simulink model "transmitter"  (R2020b)
settings: Solver=FixedStepDiscrete  StartTime=0.0  StopTime=100000  RelTol=1e-3
undefined symbols (not defined in the file): message
libraries: hdlsllib x24, simulink x11, dspmlti4 x2, whdlio x1
(part 2 of 2)

== matlab function transmitter/tran_dut/ldpc_encoder/address_calculator/addresses ==
  settings: fimath=fimath('RoundingMethod', 'Floor','OverflowAction', 'Wrap','ProductMode', 'FullPrecision', 'SumMode', 'FullPrecision')
  data: slot input; counter input; q_factor input; addresses output; bit_addresses parameter uint16; num_parity_bits parameter
function addresses = address_generator(slot, counter, q_factor, bit_addresses, num_parity_bits)
%#codegen 

addresses = fi(zeros(12, 1), 0, 14, 0);

coder.hdl.loopspec('unroll');
% Get the new parity address
for i = 1:12
    tmp = fi(16200, 0, 15, 0);
    if bit_addresses(slot, i) < 16200
        % Compute the new address
        tmp = fi(bit_addresses(slot, i) + counter*q_factor, 0, 15, 0);
        % Get the modulo 16200 if necessary.
        if tmp >= num_parity_bits
            tmp = fi(tmp - num_parity_bits, 0, 15, 0);
        end
    end
    addresses(i) = fi(tmp, 0, 14, 0);
end

== matlab function transmitter/tran_dut/ldpc_encoder/select_address ==
  settings: fimath=fimath('RoundingMethod', 'Floor','OverflowAction', 'Wrap','ProductMode', 'FullPrecision', 'SumMode', 'FullPrecision')
  data: addresses input; a1 output; a2 output; a3 output; a4 output; a5 output; a6 output; a7 output; a8 output; a9 output; a10 output; a11 output; a12 output
function [a1,a2,a3,a4,a5,a6,...
          a7,a8,a9,a10,a11,a12] = select(addresses)
%#codegen

a1 = addresses(1);
a2 = addresses(2);
a3 = addresses(3);
a4 = addresses(4);
a5 = addresses(5);
a6 = addresses(6);
a7 = addresses(7);
a8 = addresses(8);
a9 = addresses(9);
a10 = addresses(10);
a11 = addresses(11);
a12 = addresses(12);

== matlab function transmitter/tran_dut/bch_encoder/output_mask ==
  settings: fimath=fimath('RoundingMethod', 'Floor','OverflowAction', 'Wrap','ProductMode', 'FullPrecision', 'SumMode', 'FullPrecision')
  data: bit_in input; mask output
function mask = bitmask(bit_in)
%#codegen

if bit_in
    mask = fi(ones(192, 1), 0, 1, 0);
else
    mask = fi(zeros(192, 1), 0, 1, 0);
end

== matlab function transmitter/tran_dut/bch_encoder/p2s ==
  settings: fimath=fimath('RoundingMethod', 'Floor','OverflowAction', 'Wrap','ProductMode', 'FullPrecision', 'SumMode', 'FullPrecision')
  data: parallel_in input; serial_out output fixdt(0,1,0); enable input; input_length parameter uint16; valid output
function [serial_out, valid] = p2s_buffer(parallel_in, enable, input_length)
%#codegen

state_iddle    = 0;
state_reading  = 1;

persistent moore_state_machine;
if isempty(moore_state_machine)
    moore_state_machine = fi(0, 0, 1, 0);
end

persistent counter;
if isempty(counter)
    counter = fi(1, 0, 16, 0);
end

persistent buffer;
if isempty(buffer)
    buffer = parallel_in;
end

switch moore_state_machine
    case state_iddle
        serial_out = fi(0, 0, 1, 0);
        valid      = fi(0, 0, 1, 0);
        if enable
            moore_state_machine(1) = state_reading;
            buffer = parallel_in;
            serial_out          = buffer(input_length+1-counter);
            valid      = fi(1, 0, 1, 0);
            counter             = fi(counter + 1, 0, 16, 0);
        end
    case state_reading
        serial_out = buffer(input_length+1-counter);
        counter    = fi(counter + 1, 0, 16, 0);
        valid      = fi(1, 0, 1, 0);
        if(counter > input_length)
            counter = fi(1, 0, 16, 0);
            moore_state_machine(1) = state_iddle;
        end
    otherwise
        serial_out = fi(0, 0, 1, 0);
        valid      = fi(0, 0, 1, 0);
end

== matlab function transmitter/tran_dut/bch_encoder/registers ==
  settings: fimath=fimath('RoundingMethod', 'Floor','OverflowAction', 'Wrap','ProductMode', 'FullPrecision', 'SumMode', 'FullPrecision')
  data: registers_in input; out output fixdt(0,1,0) size=1; registers_out output fixdt(0,1,0) size=192
function [out, registers_out] = state_registers(registers_in)
%#codegen

persistent lfsr;
if isempty(lfsr)
    lfsr = fi(zeros(192, 1), 0, 1, 0);
else
    lfsr = registers_in;
end
out = lfsr(192);
registers_out = lfsr;

== matlab function transmitter/tran_dut/bch_encoder/shift_and_xor ==
  settings: fimath=fimath('RoundingMethod', 'Floor','OverflowAction', 'Wrap','ProductMode', 'FullPrecision', 'SumMode', 'FullPrecision')
  data: input_bit input; registers_out output fixdt(0,1,0); registers_in input; flag input
function registers_out = shift_and_xor(input_bit, registers_in, flag)
%#codegen

buffer = [input_bit; registers_in(1:192-1)];
registers_out = fi(xor(buffer, flag), 0, 1, 0);
